simulink library "libbha_kinetic_cc"  (R2013b)
settings: Solver=FixedStepDiscrete  StartTime=0.0  StopTime=Inf  FixedStep=0.004  RelTol=1e-3
PostLoadFcn:
  | , if any(exist('dsrtsu_mdlpostloadfcn', 'file') == [2, 3, 6]), try dsrtsu_mdlpostloadfcn('Execute', bdroot); catch fprintf('Error in PostLoadFcn (dsrtsu_mdlpostloadfcn) for model "%s":\n %s\n', bdroot, lasterr); end, end,
libraries: libbha_parts_bellows x2
(part 3 of 4)

== matlab function libbha_kinetic_cc/lib_kinm_ext ==
  data: q input size=[9,1]; dq input size=[9,1]; H_1b_w input size=[4,4]; PAR_ell_ib input size=[3,1]; PAR_ell_ih input size=[3,1]; PAR_r_Bi input size=[3,1]; H_1h_w output size=[4,4]; H_2h_w output size=[4,4]; H_3h_w output size=[4,4]; dHdq_1h_w output size=[36,4]; dHdq_2h_w output size=[36,4]; dHdq_3h_w output size=[36,4]; dHPdq_1h_w output size=[36,4]; dHPdq_2h_w output size=[36,4]; dHPdq_3h_w output size=[36,4]; r_Bik_1h output size=[4,3]; r_Bik_2h output size=[4,3]; r_Bik_3h output size=[4,3]
% Kinetic Simulation
function [H_1h_w, H_2h_w, H_3h_w, dHdq_1h_w, dHdq_2h_w, dHdq_3h_w, dHPdq_1h_w, dHPdq_2h_w, dHPdq_3h_w, r_Bik_1h, r_Bik_2h, r_Bik_3h] =  ksim_ext(q,dq, H_1b_w, PAR_ell_ib, PAR_ell_ih, PAR_r_Bi)

  
    
    % Änderungen zut alten Version:
    % - Rückrechnung mit Offsets der 4. Dimension der Homogenen Transformation (HOxx)
    % - richtige Saturierung des Ausgangsdrucks (optional)
    % - Tensordarstellung vermieden (Vektoren oder Matrizen sofern möglich), daher auch mehr getrennte Variablen
    % - Zusammenfassung bei Berechnungen unter Ausnutzung von 0-Einträgen (schwerer lesbar und weniger allgemein, dafür schneller zu rechnen)


%% Zustands- und Ableitungsberechnung der Homogenen Transformationen
    
    k                 = [ calc_k_i(q(1), q(2), q(3), PAR_r_Bi(1));
                          calc_k_i(q(4), q(5), q(6), PAR_r_Bi(2));
                          calc_k_i(q(7), q(8), q(9), PAR_r_Bi(3)) ];
    
    dkdq_S1              = calc_dkdq_i(q(1), q(2), q(3), PAR_r_Bi(1));
    dkdq_S2              = calc_dkdq_i(q(4), q(5), q(6), PAR_r_Bi(2));
    dkdq_S3              = calc_dkdq_i(q(7), q(8), q(9), PAR_r_Bi(3));
	
	d2kdqdq_S1 	  = calc_d2kdqdq_i(q(1), q(2), q(3), PAR_r_Bi(1));
	d2kdqdq_S2 	  = calc_d2kdqdq_i(q(4), q(5), q(6), PAR_r_Bi(2));
	d2kdqdq_S3 	  = calc_d2kdqdq_i(q(7), q(8), q(9), PAR_r_Bi(3));
    
    % Relative Homogene Transformation und dessen Ableitung im lokalen Sektions-KoSy    
	[H_1h_1b, H_1b1, H_1h1] = calc_H_ih_ib(k(1), k(2), k(3), PAR_ell_ib(1), PAR_ell_ih(1));
    [H_2h_2b, H_2b2, H_2h2] = calc_H_ih_ib(k(4), k(5), k(6), PAR_ell_ib(2), PAR_ell_ih(2));
    [H_3h_3b, H_3b3, H_3h3] = calc_H_ih_ib(k(7), k(8), k(9), PAR_ell_ib(3), PAR_ell_ih(3));
    
    [dHdq_1h_1b, dHdk_1h_1b] = calc_dHdq_ih_ib(k(1), k(2), k(3), dkdq_S1, H_1b1, H_1h1);
    [dHdq_2h_2b, dHdk_2h_2b] = calc_dHdq_ih_ib(k(4), k(5), k(6), dkdq_S2, H_2b2, H_2h2);
    [dHdq_3h_3b, dHdk_3h_3b] = calc_dHdq_ih_ib(k(7), k(8), k(9), dkdq_S3, H_3b3, H_3h3);
	
   %[d2Hdqdq_1h_1b, d2Hdkdk_1h_1b] = calc_d2Hdqdq_ih_ib(k(1), k(2), k(3), dkdq_S1, d2kdqdq_S1, dHdk_1h_1b, H_1b1, H_1h1);
   %[d2Hdqdq_2h_2b, d2Hdkdk_2h_2b] = calc_d2Hdqdq_ih_ib(k(4), k(5), k(6), dkdq_S2, d2kdqdq_S2, dHdk_2h_2b, H_2b2, H_2h2);
   %[d2Hdqdq_3h_3b, d2Hdkdk_3h_3b] = calc_d2Hdqdq_ih_ib(k(7), k(8), k(9), dkdq_S3, d2kdqdq_S3, dHdk_3h_3b, H_3b3, H_3h3);
    [d2Hdqdq_1h_1b, ~            ] = calc_d2Hdqdq_ih_ib(k(1), k(2), k(3), dkdq_S1, d2kdqdq_S1, dHdk_1h_1b, H_1b1, H_1h1);
	[d2Hdqdq_2h_2b, ~            ] = calc_d2Hdqdq_ih_ib(k(4), k(5), k(6), dkdq_S2, d2kdqdq_S2, dHdk_2h_2b, H_2b2, H_2h2);
	[d2Hdqdq_3h_3b, ~            ] = calc_d2Hdqdq_ih_ib(k(7), k(8), k(9), dkdq_S3, d2kdqdq_S3, dHdk_3h_3b, H_3b3, H_3h3);
    
    % Absolute Homogene Transformation und dessen Ableitung im Welt-KoSy
    H_1h_w = H_1b_w * H_1h_1b;
    H_2h_w = H_1h_w * H_2h_2b;
    H_3h_w = H_2h_w * H_3h_3b; 
    
    dHdq_1h_w = zeros(4*9,4); % 4x4 Matrix abgeleitet nach 9 Zuständen q_i. H1 nach Zuständen 4..9 ist 0.
    dHdq_2h_w = zeros(4*9,4); % 4x4 Matrix abgeleitet nach 9 Zuständen q_i. H2 nach Zuständen 7..9 ist 0.
    dHdq_3h_w = zeros(4*9,4); % 4x4 Matrix abgeleitet nach 9 Zuständen q_i. 
    dHdq_1h_w((1:12)   ,:) = MM(H_1b_w,dHdq_1h_1b);
    dHdq_2h_w((1:12)   ,:) = MM(dHdq_1h_w(1:12,:),H_2h_2b);
    dHdq_2h_w((1:12)+12,:) = MM(H_1h_w,dHdq_2h_2b);
    dHdq_3h_w((1:24)   ,:) = MM(dHdq_2h_w(1:24,:),H_3h_3b);
    dHdq_3h_w((1:12)+24,:) = MM(H_2h_w,dHdq_3h_3b);
	
	d2Hdqdq_1h_w = zeros(4*9,4*9);
	d2Hdqdq_2h_w = zeros(4*9,4*9);
	d2Hdqdq_3h_w = zeros(4*9,4*9);
	d2Hdqdq_1h_w((1:12)   ,(1:12)   ) = MM(H_1b_w, d2Hdqdq_1h_1b);
	d2Hdqdq_2h_w((1:12)   ,(1:12)   ) = MM(d2Hdqdq_1h_w(1:12,1:12), H_2h_2b); % Quadrat innen
	d2Hdqdq_2h_w((1:12)   ,(1:4 )+12) = MM(dHdq_1h_w(1:12,:), dHdq_2h_2b(1:4 ,:)); % Blöcke Spalte rechts
	d2Hdqdq_2h_w((1:12)   ,(5:8 )+12) = MM(dHdq_1h_w(1:12,:), dHdq_2h_2b(5:8 ,:));
	d2Hdqdq_2h_w((1:12)   ,(9:12)+12) = MM(dHdq_1h_w(1:12,:), dHdq_2h_2b(9:12,:));
	d2Hdqdq_2h_w((1:12)+12,(1:12)+12) = MM(H_1h_w, d2Hdqdq_2h_2b); % Block Diagonal
	d2Hdqdq_2h_w((1:12)+12,(1:12)   ) = transpose4x4(d2Hdqdq_2h_w(1:12,(1:12)+12)); % Blöcke Zeile unten
	d2Hdqdq_3h_w((1:24)   ,(1:24)   ) = MM(d2Hdqdq_2h_w(1:24,1:24), H_3h_3b); % Quadrat innen
	d2Hdqdq_3h_w((1:24)   ,(1:4 )+24) = MM(dHdq_2h_w(1:24,:), dHdq_3h_3b(1:4 ,:)); % Blöcke Spalte rechts
	d2Hdqdq_3h_w((1:24)   ,(5:8 )+24) = MM(dHdq_2h_w(1:24,:), dHdq_3h_3b(5:8 ,:));
	d2Hdqdq_3h_w((1:24)   ,(9:12)+24) = MM(dHdq_2h_w(1:24,:), dHdq_3h_3b(9:12,:));
	d2Hdqdq_3h_w((1:12)+24,(1:12)+24) = MM(H_2h_w, d2Hdqdq_3h_3b); % Block Diagonal
	d2Hdqdq_3h_w((1:12)+24,(1:24)   ) = transpose4x4(d2Hdqdq_3h_w(1:24,(1:12)+24)); % Blöcke Zeile unten
	
	% Funktionen der Zeitableitung (HP)
	%HP_1h_w = calc_HP(dHdq_1h_w, dq); %zeros(4*9,4);
	%HP_2h_w = calc_HP(dHdq_2h_w, dq);
	%HP_3h_w = calc_HP(dHdq_3h_w, dq);
	
	dHPdq_1h_w = calc_dHPdq(d2Hdqdq_1h_w, dq); %zeros(4*9,4);
	dHPdq_2h_w = calc_dHPdq(d2Hdqdq_2h_w, dq);
	dHPdq_3h_w = calc_dHPdq(d2Hdqdq_3h_w, dq);
	
%% Kinetische Vorwärtsrechnung

    %r_S1_1h = [0;0;0;1];
    %r_S2_2h = [0;0;0;1];
    %r_S3_3h = [0;0;0;1];
    
    r_Bik_1h = [ PAR_r_Bi(1), -PAR_r_Bi(1)/2,         -PAR_r_Bi(1)/2;
				 0,            sqrt(3)/2*PAR_r_Bi(1),  -sqrt(3)/2*PAR_r_Bi(1)  
                 0, 0, 0; 1, 1, 1 ];
    r_Bik_2h = [ PAR_r_Bi(2), -PAR_r_Bi(2)/2,         -PAR_r_Bi(2)/2;
				 0,            sqrt(3)/2*PAR_r_Bi(2),  -sqrt(3)/2*PAR_r_Bi(2)  
                 0, 0, 0; 1, 1, 1 ];
    r_Bik_3h = [ PAR_r_Bi(3), -PAR_r_Bi(3)/2,         -PAR_r_Bi(3)/2;
				 0,            sqrt(3)/2*PAR_r_Bi(3),  -sqrt(3)/2*PAR_r_Bi(3)  
                 0, 0, 0; 1, 1, 1 ];

end

% ##################### Hilfsfunktionen #####################

%%  Konfigurationszustand k = [phi, kappa, ell]^T 

%  Konfigurationszustand einer Sektion 
function [k_i] = calc_k_i(q1,q2,q3, d)
    % Input:
    %   - qi = [ell_i1, ell_i2, ell_i3]^T       Aktorzustand
    %   - d                                     Radialer Abstand der Aktorsymmetrielinie  
    %
    % Output:
    %   - ki   [3 x 1]                          Konfigurationszustand 

    % Vermeidung Singularität
    qist_eps  = 1e-15;
    qist      = q1.^2 + q2.^2 + q3.^2 - q1.*q2 - q1.*q3 - q2.*q3;
    while (qist<qist_eps)
        q1      = q1 - 5e-8;
        qist  = q1.^2 + q2.^2 + q3.^2 - q1.*q2 - q1.*q3 - q2.*q3;
    end

    % Substitutionen
    q_sum   = q1 + q2 + q3;
    
    % Konfigurationszustand
    mphi    = atan2(sqrt(0.3e1) * (q3-q2) , (q2+q3 - 2*q1));
    mkappa  = 2.0 * sqrt(qist) / (d*q_sum);
    mell    = (q1 + q2 + q3)/3.0;
    
    k_i = [mphi;
           mkappa;
           mell];
end

% Partielle Ableitung 1. Ordnung nach q
function [dkdq_i] = calc_dkdq_i(q1,q2,q3, d)

    % Input:
	%   - qi = [ell_i1, ell_i2, ell_i3]^T       Aktorzustand
    %   - d                                     Radialer Abstand der Aktorsymmetrielinie
	%
	% Output:
	%   - dkdq_i   [3 x 3]                      Partielle Ableitung von Konfigurationszuständen ki nach Aktorzuständen qi 
 
    % Vermeidung Singularität
    qist_eps  = 1e-15;
    qist      = q1.^2 + q2.^2 + q3.^2 - q1.*q2 - q1.*q3 - q2.*q3;
    while (qist<qist_eps)
        q1      = q1-5e-8;
        qist  = q1.^2 + q2.^2 + q3.^2 - q1*q2 - q1*q3 - q2*q3;
    end

    % Substitutionen
    q_sum   = q1 + q2 + q3;

    % Ableitungen
    dkdq_i = zeros(3, 3);
    
    % dk1_dqb
    mdphi_dq1 =  sqrt(3.0) * ( q3 - q2) / qist / 2.0;
    mdphi_dq2 =  sqrt(3.0) * (-q3 + q1) / qist / 2.0;
    mdphi_dq3 = -sqrt(3.0) * (-q2 + q1) / qist / 2.0;
    
    dkdq_i(1, :) = [mdphi_dq1, mdphi_dq2, mdphi_dq3];
    
    % dk2_dqb
    mdkappa_dq1 =  3 * ( q2*q1 - q2^2  + q3*q1 - q3^2) / sqrt(qist) / d / q_sum^2;
    mdkappa_dq2 = -3 * (-q2*q1 - q2*q3 + q3^2  + q1^2) / sqrt(qist) / d / q_sum^2;
    mdkappa_dq3 = -3 * ( q2^2  - q2*q3 - q3*q1 + q1^2) / sqrt(qist) / d / q_sum^2;
    
    dkdq_i(2, :) = [mdkappa_dq1, mdkappa_dq2, mdkappa_dq3];
    
    % dk3_dqb
    mdell_dq1 = 1.0/3.0;
    mdell_dq2 = 1.0/3.0;
    mdell_dq3 = 1.0/3.0;
    
    dkdq_i(3, :) = [mdell_dq1, mdell_dq2, mdell_dq3];
end

function [d2kdqdq_i] = calc_d2kdqdq_i(q1,q2,q3, d)
% Input:
%   - qi = [ell_i1, ell_i2, ell_i3]^T       Aktorzustand
%
% Output:
%   - d2kdqdq_S1   [3*dim_qi x dim_qi]   Partielle Ableitung 2.Ord. von allen Konfigurationszuständen ki nach allen Aktorzuständen qi 
 
    % Vermeidung Singularität
    q_dist_eps  = 1e-15;
    q_dist      = q1 ^ 2 + q2 ^ 2 + q3 ^ 2 - q1 * q2 - q1 * q3 - q2 * q3;
    while (q_dist<q_dist_eps)
        q1      = q1-5e-8;
        q_dist  = q1 ^ 2 + q2 ^ 2 + q3 ^ 2 - q1 * q2 - q1 * q3 - q2 * q3;
    end

    % Substitutionen
    q_sum   = q1 + q2 + q3;

    % Ableitungen
    d2kdqdq_i = zeros(3*3, 3);
    
    % d2k1_dqbdqc
    mddphi_dq1dq1 = -sqrt(0.3e1) * (q3 - q2) / q_dist ^ 2 * (-q2 - q3 + 2 * q1) / 0.2e1;
    mddphi_dq1dq2 = -sqrt(0.3e1) * (-q2 ^ 2 + 2 * q2 * q3 - 2 * q3 * q1 + q1 ^ 2) / q_dist ^ 2 / 0.2e1;
    mddphi_dq1dq3 = sqrt(0.3e1) * (2 * q2 * q3 - 2 * q2 * q1 - q3 ^ 2 + q1 ^ 2) / q_dist ^ 2 / 0.2e1;
    
    mddphi_dq2dq1 = mddphi_dq1dq2;
    mddphi_dq2dq2 = sqrt(0.3e1) * (-q3 + q1) * (-2 * q2 + q3 + q1) / q_dist ^ 2 / 0.2e1;
    mddphi_dq2dq3 = -sqrt(0.3e1) * (q2 ^ 2 - 2 * q2 * q1 - q3 ^ 2 + 2 * q3 * q1) / q_dist ^ 2 / 0.2e1;
    
    mddphi_dq3dq1 = mddphi_dq1dq3;
    mddphi_dq3dq2 = mddphi_dq2dq3;
    mddphi_dq3dq3 = -sqrt(0.3e1) * (-q2 + q1) * (q2 - 2 * q3 + q1) / q_dist ^ 2 / 0.2e1;
    
    d2kdqdq_i([1, 4, 7], 1) = [mddphi_dq1dq1, mddphi_dq2dq1, mddphi_dq3dq1];
    d2kdqdq_i([1, 4, 7], 2) = [mddphi_dq1dq2, mddphi_dq2dq2, mddphi_dq3dq2];
    d2kdqdq_i([1, 4, 7], 3) = [mddphi_dq1dq3, mddphi_dq2dq3, mddphi_dq3dq3];
    
    % dk2_dqbdqc
    mddkappa_dq1dq1 = -0.3e1 / 0.2e1 * (-6 * q2 * q1 ^ 2 * q3 + 6 * q2 * q1 * q3 ^ 2 + 6 * q2 ^ 2 * q1 * q3 - 9 * q2 ^ 2 * q1 ^ 2 - 5 * q2 ^ 4 - 5 * q3 ^ 4 + 4 * q3 ^ 3 * q2 + 6 * q2 ^ 3 * q1 + 4 * q2 * q1 ^ 3 + 4 * q2 ^ 3 * q3 - 6 * q2 ^ 2 * q3 ^ 2 - 9 * q3 ^ 2 * q1 ^ 2 + 6 * q3 ^ 3 * q1 + 4 * q3 * q1 ^ 3) * (q_dist ^ (-0.3e1 / 0.2e1)) / d / (q_sum ^ 3);
    mddkappa_dq1dq2 = 0.3e1 / 0.2e1 * (2 * q2 ^ 4 + 3 * q3 ^ 4 + 3 * q2 * q1 ^ 2 * q3 + 3 * q2 ^ 2 * q1 * q3 - 3 * q2 * q1 * q3 ^ 2 + 6 * q2 ^ 2 * q1 ^ 2 - 7 * q2 ^ 3 * q1 - 7 * q2 * q1 ^ 3 - 3 * q2 ^ 3 * q3 + 9 * q2 ^ 2 * q3 ^ 2 - 3 * q3 * q1 ^ 3 + 9 * q3 ^ 2 * q1 ^ 2 - 7 * q3 ^ 3 * q2 - 7 * q3 ^ 3 * q1 + 2 * q1 ^ 4) * (q_dist ^ (-0.3e1 / 0.2e1)) / d / (q_sum ^ 3);
    mddkappa_dq1dq3 = 0.3e1 / 0.2e1 * (3 * q2 ^ 4 + 2 * q3 ^ 4 + 3 * q2 * q1 ^ 2 * q3 - 3 * q2 ^ 2 * q1 * q3 + 3 * q2 * q1 * q3 ^ 2 + 9 * q2 ^ 2 * q1 ^ 2 - 7 * q2 ^ 3 * q1 - 3 * q2 * q1 ^ 3 - 7 * q2 ^ 3 * q3 + 9 * q2 ^ 2 * q3 ^ 2 - 7 * q3 * q1 ^ 3 + 6 * q3 ^ 2 * q1 ^ 2 - 3 * q3 ^ 3 * q2 - 7 * q3 ^ 3 * q1 + 2 * q1 ^ 4) * (q_dist ^ (-0.3e1 / 0.2e1)) / d / (q_sum ^ 3);
    
    mddkappa_dq2dq1 = mddkappa_dq1dq2;
    mddkappa_dq2dq2 = 0.3e1 / 0.2e1 * (5 * q3 ^ 4 - 6 * q2 * q1 ^ 2 * q3 + 6 * q2 ^ 2 * q1 * q3 - 6 * q2 * q1 * q3 ^ 2 + 9 * q2 ^ 2 * q1 ^ 2 - 4 * q2 ^ 3 * q1 - 6 * q2 * q1 ^ 3 - 4 * q2 ^ 3 * q3 + 9 * q2 ^ 2 * q3 ^ 2 - 4 * q3 * q1 ^ 3 + 6 * q3 ^ 2 * q1 ^ 2 - 6 * q3 ^ 3 * q2 - 4 * q3 ^ 3 * q1 + 5 * q1 ^ 4) * (q_dist ^ (-0.3e1 / 0.2e1)) / d / (q_sum ^ 3);
    mddkappa_dq2dq3 = 0.3e1 / 0.2e1 * (2 * q2 ^ 4 + 2 * q3 ^ 4 - 3 * q2 * q1 ^ 2 * q3 + 3 * q2 ^ 2 * q1 * q3 + 3 * q2 * q1 * q3 ^ 2 + 9 * q2 ^ 2 * q1 ^ 2 - 3 * q2 ^ 3 * q1 - 7 * q2 ^ 3 * q3 + 6 * q2 ^ 2 * q3 ^ 2 - 7 * q2 * q3 ^ 3 - 3 * q3 ^ 3 * q1 + 9 * q3 ^ 2 * q1 ^ 2 - 7 * q1 ^ 3 * q3 - 7 * q1 ^ 3 * q2 + 3 * q1 ^ 4) * (q_dist ^ (-0.3e1 / 0.2e1)) / d / (q_sum ^ 3);

    mddkappa_dq3dq1 = mddkappa_dq1dq3;
    mddkappa_dq3dq2 = mddkappa_dq2dq3;
    mddkappa_dq3dq3 = 0.3e1 / 0.2e1 * (5 * q2 ^ 4 - 6 * q2 * q1 ^ 2 * q3 - 6 * q2 ^ 2 * q1 * q3 + 6 * q2 * q1 * q3 ^ 2 + 6 * q2 ^ 2 * q1 ^ 2 - 4 * q2 ^ 3 * q1 - 6 * q2 ^ 3 * q3 + 9 * q2 ^ 2 * q3 ^ 2 - 4 * q2 * q3 ^ 3 - 4 * q3 ^ 3 * q1 + 9 * q3 ^ 2 * q1 ^ 2 - 6 * q1 ^ 3 * q3 - 4 * q1 ^ 3 * q2 + 5 * q1 ^ 4) * (q_dist ^ (-0.3e1 / 0.2e1)) / d / (q_sum ^ 3);

    d2kdqdq_i([2, 5, 8], 1) = [mddkappa_dq1dq1, mddkappa_dq2dq1, mddkappa_dq3dq1];
    d2kdqdq_i([2, 5, 8], 2) = [mddkappa_dq1dq2, mddkappa_dq2dq2, mddkappa_dq3dq2];
    d2kdqdq_i([2, 5, 8], 3) = [mddkappa_dq1dq3, mddkappa_dq2dq3, mddkappa_dq3dq3];
    
    % dk3_dqbdqc
    % partielle Ableitungen 2. Ord von ell sind alle 0
end

%%  Homogene Transformationen 

%  Homogene Transformation 
%function [H_ih_ib] = calc_H_ih_ib(k1, k2, k3, PAR_ell_ib, PAR_ell_ih) 
function [H_ih_ib, H_im1_ib, H_ih_i] = calc_H_ih_ib(k1, k2, k3, PAR_ell_ib, PAR_ell_ih) 
    % Input:
    %   - ki = [phi, kappa, ell]^T              Konfigurationszustand
    %
    % Output:
    %   - H_i_im1   [4 x 4]                     Homogene Transformation
    
    % Vermeidung Singularität
    k2_eps = 1e-6;
    k2     = max([k2_eps, k2]);
    
    % Substitutionen
    sk1     = sin(k1);
    ck1     = cos(k1);
    sk2k3   = sin(k2 * k3);
    ck2k3   = cos(k2 * k3);
    
    % Trafo
    mHT_i_im1_11 = ck1 ^ 2 * (ck2k3 - 0.1e1) + 0.1e1;
    mHT_i_im1_12 = sk1 * ck1 * (ck2k3 - 0.1e1);
    mHT_i_im1_13 = ck1 * sk2k3;
    mHT_i_im1_14 = -ck1 * (ck2k3 - 0.1e1) / k2;
    
    mHT_i_im1_21 = sk1 * ck1 * (ck2k3 - 0.1e1);
    mHT_i_im1_22 = -ck1 ^ 2 * (ck2k3 - 0.1e1) + ck2k3;
    mHT_i_im1_23 = sk1 * sk2k3;
    mHT_i_im1_24 = -sk1 * (ck2k3 - 0.1e1) / k2;
    
    mHT_i_im1_31 = -ck1 * sk2k3;
    mHT_i_im1_32 = -sk1 * sk2k3;
    mHT_i_im1_33 = ck2k3;
    mHT_i_im1_34 = sk2k3 / k2;
    
    H_i_im1 = [mHT_i_im1_11, mHT_i_im1_12, mHT_i_im1_13, mHT_i_im1_14;
               mHT_i_im1_21, mHT_i_im1_22, mHT_i_im1_23, mHT_i_im1_24;
               mHT_i_im1_31, mHT_i_im1_32, mHT_i_im1_33, mHT_i_im1_34;
               0,            0,            0,            1            ];
           
    % Statische Begrenzungen
    H_im1_ib = eye(4);    
    H_ih_i   = eye(4);
    H_im1_ib(3,4) = PAR_ell_ib;
	H_ih_i(3,4)   = PAR_ell_ih;
    
    H_ih_ib = H_im1_ib * H_i_im1 * H_ih_i;
end

function [dHdk_i_i] = calc_dHdk_i_i(k1, k2, k3)
    % Input:
	%   - ki = [phi, kappa, ell]^T              Konfigurationszustand
	%
	% Output:
	%   - dH_i_in_im1_dka   [4*3x4]      Partielle Ableitung von H_i_in_im1 nach allen Konfigurationszuständen ki mit dim_ki=3
    
    % Vermeidung Singularität
    k2_eps = 1e-6;
    k2     = max([k2_eps, k2]);
    
    % Substitutionen
    sk1     = sin(k1);
    ck1     = cos(k1);
    sk2k3   = sin(k2 * k3);
    ck2k3   = cos(k2 * k3);
    
    dHdk_i_i = zeros(4*3, 4);
    
    % dHdk1_i_im1
    mdH_i_in_im1_dk1_11 = -2 * sk1 * ck1 * (ck2k3 - 1);
    mdH_i_in_im1_dk1_12 = 2 * ck2k3 * ck1 ^ 2 - ck2k3 - 2 * ck1 ^ 2 + 1;
    mdH_i_in_im1_dk1_13 = -sk1 * sk2k3;
    mdH_i_in_im1_dk1_14 = sk1 * (ck2k3 - 1) / k2;
    
    mdH_i_in_im1_dk1_21 = 2 * ck2k3 * ck1 ^ 2 - ck2k3 - 2 * ck1 ^ 2 + 1;
    mdH_i_in_im1_dk1_22 = 2 * sk1 * ck1 * (ck2k3 - 1);
    mdH_i_in_im1_dk1_23 = ck1 * sk2k3;
    mdH_i_in_im1_dk1_24 = -ck1 * (ck2k3 - 1) / k2;
    
    mdH_i_in_im1_dk1_31 = sk1 * sk2k3;
    mdH_i_in_im1_dk1_32 = -ck1 * sk2k3;
    mdH_i_in_im1_dk1_33 = 0;
    mdH_i_in_im1_dk1_34 = 0;
    
    dHdk_i_i(1:3,:) =         [mdH_i_in_im1_dk1_11, mdH_i_in_im1_dk1_12, mdH_i_in_im1_dk1_13, mdH_i_in_im1_dk1_14;
                               mdH_i_in_im1_dk1_21, mdH_i_in_im1_dk1_22, mdH_i_in_im1_dk1_23, mdH_i_in_im1_dk1_24;
                               mdH_i_in_im1_dk1_31, mdH_i_in_im1_dk1_32, mdH_i_in_im1_dk1_33, mdH_i_in_im1_dk1_34 ];
    
    % dHdk2_i_im1
    mdH_i_in_im1_dk2_11 = -ck1 ^ 2 * sk2k3 * k3;
    mdH_i_in_im1_dk2_12 = -sk1 * ck1 * sk2k3 * k3;
    mdH_i_in_im1_dk2_13 = ck1 * ck2k3 * k3;
    mdH_i_in_im1_dk2_14 = ck1 * (sk2k3 * k3 * k2 + ck2k3 - 1) / k2 ^ 2;
    
    mdH_i_in_im1_dk2_21 = -sk1 * ck1 * sk2k3 * k3;
    mdH_i_in_im1_dk2_22 = -sk2k3 * sk1 ^ 2 * k3;
    mdH_i_in_im1_dk2_23 = sk1 * ck2k3 * k3;
    mdH_i_in_im1_dk2_24 = sk1 * (sk2k3 * k3 * k2 + ck2k3 - 1) / k2 ^ 2;
    
    mdH_i_in_im1_dk2_31 = -ck1 * ck2k3 * k3;
    mdH_i_in_im1_dk2_32 = -sk1 * ck2k3 * k3;
    mdH_i_in_im1_dk2_33 = -sk2k3 * k3;
    mdH_i_in_im1_dk2_34 = (ck2k3 * k3 * k2 - sk2k3) / k2 ^ 2;
    
    dHdk_i_i(5:7,:) =         [mdH_i_in_im1_dk2_11, mdH_i_in_im1_dk2_12, mdH_i_in_im1_dk2_13, mdH_i_in_im1_dk2_14;
                               mdH_i_in_im1_dk2_21, mdH_i_in_im1_dk2_22, mdH_i_in_im1_dk2_23, mdH_i_in_im1_dk2_24;
                               mdH_i_in_im1_dk2_31, mdH_i_in_im1_dk2_32, mdH_i_in_im1_dk2_33, mdH_i_in_im1_dk2_34 ];
    
    % dHdk3_i_im1
    mdH_i_in_im1_dk3_11 = -ck1 ^ 2 * sk2k3 * k2;
    mdH_i_in_im1_dk3_12 = -sk1 * ck1 * sk2k3 * k2;
    mdH_i_in_im1_dk3_13 = ck1 * ck2k3 * k2;
    mdH_i_in_im1_dk3_14 = ck1 * sk2k3;
    
    mdH_i_in_im1_dk3_21 = -sk1 * ck1 * sk2k3 * k2;
    mdH_i_in_im1_dk3_22 = -sk2k3 * sk1 ^ 2 * k2;
    mdH_i_in_im1_dk3_23 = sk1 * ck2k3 * k2;
    mdH_i_in_im1_dk3_24 = sk1 * sk2k3;
    
    mdH_i_in_im1_dk3_31 = -ck1 * ck2k3 * k2;
    mdH_i_in_im1_dk3_32 = -sk1 * ck2k3 * k2;
    mdH_i_in_im1_dk3_33 = -sk2k3 * k2;
    mdH_i_in_im1_dk3_34 = ck2k3;
    
    dHdk_i_i(9:11,:) =        [mdH_i_in_im1_dk3_11, mdH_i_in_im1_dk3_12, mdH_i_in_im1_dk3_13, mdH_i_in_im1_dk3_14;
                               mdH_i_in_im1_dk3_21, mdH_i_in_im1_dk3_22, mdH_i_in_im1_dk3_23, mdH_i_in_im1_dk3_24;
                               mdH_i_in_im1_dk3_31, mdH_i_in_im1_dk3_32, mdH_i_in_im1_dk3_33, mdH_i_in_im1_dk3_34 ];
end

%function [dHdq_ih_ib, dHdk_ih_ib] = calc_dHdq_ih_ib(k1, k2, k3, dkdq_i, PAR_ell_ib, PAR_ell_ih)
function [dHdq_ih_ib, dHdk_ih_ib] = calc_dHdq_ih_ib(k1, k2, k3, dkdq_i, H_ibi, H_ihi)

    % Input:
	%   - ki = [phi, kappa, ell]^T              Konfigurationszustand
	%   - dkdq_i            [3=dim_kix3=dim_qi] Partielle Ableitung von allen Konfigurationszuständen ki nach allen Aktorzuständen qi 
	%
	% Output:
	%   - dH_i_in_im1_dqa   [4*3x4]      Partielle Ableitung von H_ih_ib nach allen Aktorzuständen qi mit dim_di = 3

    dHdq_ih_ib = zeros(4*3,4);

    % Statische Begrenzungen
    %H_im1_ib = eye(4);    
    %H_ih_i   = eye(4);
    %H_im1_ib(3,4) = PAR_ell_ib;
	%H_ih_i(3,4)   = PAR_ell_ih;
    
    % Kettenregel
    dHdk_ih_ib = calc_dHdk_i_i(k1, k2, k3);
    for j=1:3
		jm = j-1;
		%dHdq_ih_ib((1:4)+jm*4,:) = H_im1_ib * (dHdk_ih_ib(1:4,:).*dkdq_i(1,j) + dHdk_ih_ib(5:8,:).*dkdq_i(2,j) + dHdk_ih_ib(9:12,:).*dkdq_i(3,j)) * H_ih_i; % H_base * ( dHdq_i_i ) * H_head // mit dHdq_i_i = dH/dk1 * dk1/dqj + dH/dk2 * dk2/dqj + dH/dk3 * dk3/dqj
		dHdq_ih_ib((1:4)+jm*4,:) = H_ibi * (dHdk_ih_ib(1:4,:).*dkdq_i(1,j) + dHdk_ih_ib(5:8,:).*dkdq_i(2,j) + dHdk_ih_ib(9:12,:).*dkdq_i(3,j)) * H_ihi; % H_base * ( dHdq_i_i ) * H_head // mit dHdq_i_i = dH/dk1 * dk1/dqj + dH/dk2 * dk2/dqj + dH/dk3 * dk3/dqj
    end
end

function d2Hdkdk_ih_ib = calc_d2Hdkdk_ih_ib(k1, k2, k3)
% Input:
%   - ki = [phi, kappa, ell]^T              Konfigurationszustand
%
% Output
%   - d2Hdkdk_ih_ib   [4*dim_ki x 4*dim_ki]       Partielle Ableitung 2.Ord von H_i_in_im1 nach allen Konfigurationszuständen ki 
    
    % Vermeidung Singularität
    k2_eps = 1e-6;
    k2     = max([k2_eps, k2]);
    
    % Substitutionen
    sk1     = sin(k1);
    ck1     = cos(k1);
    sk2k3   = sin(k2 * k3);
    ck2k3   = cos(k2 * k3);
    
    dim_ki = 3;
    d2Hdkdk_ih_ib = zeros(4*dim_ki, 4*dim_ki);
    
% d2H_i_in_im1_dk1dk1
    mddH_i_in_im1_dk1dk1_11 = -0.4e1 * ck2k3 * ck1 ^ 2 + 0.2e1 * ck2k3 + 0.4e1 * ck1 ^ 2 - 0.2e1;
    mddH_i_in_im1_dk1dk1_12 = -0.4e1 * sk1 * ck1 * (ck2k3 - 0.1e1);
    mddH_i_in_im1_dk1dk1_13 = -ck1 * sk2k3;
    mddH_i_in_im1_dk1dk1_14 = ck1 * (ck2k3 - 0.1e1) / k2;
    
    mddH_i_in_im1_dk1dk1_21 = -0.4e1 * sk1 * ck1 * (ck2k3 - 0.1e1);
    mddH_i_in_im1_dk1dk1_22 = 0.4e1 * ck2k3 * ck1 ^ 2 - 0.2e1 * ck2k3 - 0.4e1 * ck1 ^ 2 + 0.2e1;
    mddH_i_in_im1_dk1dk1_23 = -sk1 * sk2k3;
    mddH_i_in_im1_dk1dk1_24 = sk1 * (ck2k3 - 0.1e1) / k2;
    
    mddH_i_in_im1_dk1dk1_31 = ck1 * sk2k3;
    mddH_i_in_im1_dk1dk1_32 = sk1 * sk2k3;
    mddH_i_in_im1_dk1dk1_33 = 0;
    mddH_i_in_im1_dk1dk1_34 = 0;
    
    d2Hdkdk_ih_ib(1:3, 1:4)       = [mddH_i_in_im1_dk1dk1_11, mddH_i_in_im1_dk1dk1_12, mddH_i_in_im1_dk1dk1_13, mddH_i_in_im1_dk1dk1_14;
                                           mddH_i_in_im1_dk1dk1_21, mddH_i_in_im1_dk1dk1_22, mddH_i_in_im1_dk1dk1_23, mddH_i_in_im1_dk1dk1_24;
                                           mddH_i_in_im1_dk1dk1_31, mddH_i_in_im1_dk1dk1_32, mddH_i_in_im1_dk1dk1_33, mddH_i_in_im1_dk1dk1_34 ]; 
    
    
    % d2H_i_in_im1_dk2dk2
    mddH_i_in_im1_dk2dk2_11 = -ck1 ^ 2 * ck2k3 * k3 ^ 2;
    mddH_i_in_im1_dk2dk2_12 = -sk1 * ck1 * ck2k3 * k3 ^ 2;
    mddH_i_in_im1_dk2dk2_13 = -ck1 * sk2k3 * k3 ^ 2;
    mddH_i_in_im1_dk2dk2_14 = -ck1 * (-ck2k3 * k3 ^ 2 * k2 ^ 2 + 0.2e1 * sk2k3 * k3 * k2 + 0.2e1 * ck2k3 - 0.2e1) / k2 ^ 3;
    
    mddH_i_in_im1_dk2dk2_21 = -sk1 * ck1 * ck2k3 * k3 ^ 2;
    mddH_i_in_im1_dk2dk2_22 = -ck2k3 * k3 ^ 2 * sk1 ^ 2;
    mddH_i_in_im1_dk2dk2_23 = -sk1 * sk2k3 * k3 ^ 2;
    mddH_i_in_im1_dk2dk2_24 = -sk1 * (-ck2k3 * k3 ^ 2 * k2 ^ 2 + 0.2e1 * sk2k3 * k3 * k2 + 0.2e1 * ck2k3 - 0.2e1) / k2 ^ 3;
    
    mddH_i_in_im1_dk2dk2_31 = ck1 * sk2k3 * k3 ^ 2;
    mddH_i_in_im1_dk2dk2_32 = sk1 * sk2k3 * k3 ^ 2;
    mddH_i_in_im1_dk2dk2_33 = -ck2k3 * k3 ^ 2;
    mddH_i_in_im1_dk2dk2_34 = -(sk2k3 * k3 ^ 2 * k2 ^ 2 + 0.2e1 * ck2k3 * k3 * k2 - 0.2e1 * sk2k3) / k2 ^ 3;
    
    d2Hdkdk_ih_ib(5:7, 5:8)       = [mddH_i_in_im1_dk2dk2_11, mddH_i_in_im1_dk2dk2_12, mddH_i_in_im1_dk2dk2_13, mddH_i_in_im1_dk2dk2_14;
                                           mddH_i_in_im1_dk2dk2_21, mddH_i_in_im1_dk2dk2_22, mddH_i_in_im1_dk2dk2_23, mddH_i_in_im1_dk2dk2_24;
                                           mddH_i_in_im1_dk2dk2_31, mddH_i_in_im1_dk2dk2_32, mddH_i_in_im1_dk2dk2_33, mddH_i_in_im1_dk2dk2_34 ]; 
                                       
    % d2H_i_in_im1_dk3dk3
    mddH_i_in_im1_dk3dk3_11 = -ck1 ^ 2 * ck2k3 * k2 ^ 2;
    mddH_i_in_im1_dk3dk3_12 = -sk1 * ck1 * ck2k3 * k2 ^ 2;
    mddH_i_in_im1_dk3dk3_13 = -ck1 * sk2k3 * k2 ^ 2;
    mddH_i_in_im1_dk3dk3_14 = ck1 * ck2k3 * k2;
    
    mddH_i_in_im1_dk3dk3_21 = -sk1 * ck1 * ck2k3 * k2 ^ 2;
    mddH_i_in_im1_dk3dk3_22 = -ck2k3 * k2 ^ 2 * sk1 ^ 2;
    mddH_i_in_im1_dk3dk3_23 = -sk1 * sk2k3 * k2 ^ 2;
    mddH_i_in_im1_dk3dk3_24 = sk1 * ck2k3 * k2;
    
    mddH_i_in_im1_dk3dk3_31 = ck1 * sk2k3 * k2 ^ 2;
    mddH_i_in_im1_dk3dk3_32 = sk1 * sk2k3 * k2 ^ 2;
    mddH_i_in_im1_dk3dk3_33 = -ck2k3 * k2 ^ 2;
    mddH_i_in_im1_dk3dk3_34 = -sk2k3 * k2;
    
    d2Hdkdk_ih_ib(9:11, 9:12)     = [mddH_i_in_im1_dk3dk3_11, mddH_i_in_im1_dk3dk3_12, mddH_i_in_im1_dk3dk3_13, mddH_i_in_im1_dk3dk3_14;
                                           mddH_i_in_im1_dk3dk3_21, mddH_i_in_im1_dk3dk3_22, mddH_i_in_im1_dk3dk3_23, mddH_i_in_im1_dk3dk3_24;
                                           mddH_i_in_im1_dk3dk3_31, mddH_i_in_im1_dk3dk3_32, mddH_i_in_im1_dk3dk3_33, mddH_i_in_im1_dk3dk3_34 ]; 
                                       
    % d2H_i_in_im1_dk1dk2 = d2H_i_in_im1_dk2dk1
    mddH_i_in_im1_dk1dk2_11 = 0.2e1 * sk1 * ck1 * sk2k3 * k3;
    mddH_i_in_im1_dk1dk2_12 = -sk2k3 * k3 * (0.2e1 * ck1 ^ 2 - 0.1e1);
    mddH_i_in_im1_dk1dk2_13 = -sk1 * ck2k3 * k3;
    mddH_i_in_im1_dk1dk2_14 = -sk1 * (sk2k3 * k3 * k2 + ck2k3 - 0.1e1) / k2 ^ 2;
    
    mddH_i_in_im1_dk1dk2_21 = -sk2k3 * k3 * (0.2e1 * ck1 ^ 2 - 0.1e1);
    mddH_i_in_im1_dk1dk2_22 = -0.2e1 * sk1 * ck1 * sk2k3 * k3;
    mddH_i_in_im1_dk1dk2_23 = ck1 * ck2k3 * k3;
    mddH_i_in_im1_dk1dk2_24 = ck1 * (sk2k3 * k3 * k2 + ck2k3 - 0.1e1) / k2 ^ 2;
    
    mddH_i_in_im1_dk1dk2_31 = sk1 * ck2k3 * k3;
    mddH_i_in_im1_dk1dk2_32 = -ck1 * ck2k3 * k3;
    mddH_i_in_im1_dk1dk2_33 = 0;
    mddH_i_in_im1_dk1dk2_34 = 0;
    
    d2Hdkdk_ih_ib(1:3, 5:8)       = [mddH_i_in_im1_dk1dk2_11, mddH_i_in_im1_dk1dk2_12, mddH_i_in_im1_dk1dk2_13, mddH_i_in_im1_dk1dk2_14;
                                           mddH_i_in_im1_dk1dk2_21, mddH_i_in_im1_dk1dk2_22, mddH_i_in_im1_dk1dk2_23, mddH_i_in_im1_dk1dk2_24;
                                           mddH_i_in_im1_dk1dk2_31, mddH_i_in_im1_dk1dk2_32, mddH_i_in_im1_dk1dk2_33, mddH_i_in_im1_dk1dk2_34 ]; 
    d2Hdkdk_ih_ib(5:7, 1:4) = d2Hdkdk_ih_ib(1:3, 5:8);
    
    % d2H_i_in_im1_dk1dk3 = d2H_i_in_im1_dk3dk1
    mddH_i_in_im1_dk1dk3_11 = 0.2e1 * sk1 * ck1 * sk2k3 * k2;
    mddH_i_in_im1_dk1dk3_12 = -sk2k3 * k2 * (0.2e1 * ck1 ^ 2 - 0.1e1);
    mddH_i_in_im1_dk1dk3_13 = -sk1 * ck2k3 * k2;
    mddH_i_in_im1_dk1dk3_14 = -sk1 * sk2k3;
    
    mddH_i_in_im1_dk1dk3_21 = -sk2k3 * k2 * (0.2e1 * ck1 ^ 2 - 0.1e1);
    mddH_i_in_im1_dk1dk3_22 = -0.2e1 * sk1 * ck1 * sk2k3 * k2;
    mddH_i_in_im1_dk1dk3_23 = ck1 * ck2k3 * k2;
    mddH_i_in_im1_dk1dk3_24 = ck1 * sk2k3;
    
    mddH_i_in_im1_dk1dk3_31 = sk1 * ck2k3 * k2;
    mddH_i_in_im1_dk1dk3_32 = -ck1 * ck2k3 * k2;
    mddH_i_in_im1_dk1dk3_33 = 0;
    mddH_i_in_im1_dk1dk3_34 = 0;
    
    d2Hdkdk_ih_ib(1:3, 9:12)      = [mddH_i_in_im1_dk1dk3_11, mddH_i_in_im1_dk1dk3_12, mddH_i_in_im1_dk1dk3_13, mddH_i_in_im1_dk1dk3_14;
                                           mddH_i_in_im1_dk1dk3_21, mddH_i_in_im1_dk1dk3_22, mddH_i_in_im1_dk1dk3_23, mddH_i_in_im1_dk1dk3_24;
                                           mddH_i_in_im1_dk1dk3_31, mddH_i_in_im1_dk1dk3_32, mddH_i_in_im1_dk1dk3_33, mddH_i_in_im1_dk1dk3_34 ]; 
    d2Hdkdk_ih_ib(9:11, 1:4) = d2Hdkdk_ih_ib(1:3, 9:12);
    
    % d2H_i_in_im1_dk2dk3 = d2H_i_in_im1_dk3dk2
    mddH_i_in_im1_dk2dk3_11 = -ck1 ^ 2 * (ck2k3 * k3 * k2 + sk2k3);
    mddH_i_in_im1_dk2dk3_12 = -sk1 * ck1 * (ck2k3 * k3 * k2 + sk2k3);
    mddH_i_in_im1_dk2dk3_13 = ck1 * (-sk2k3 * k3 * k2 + ck2k3);
    mddH_i_in_im1_dk2dk3_14 = ck1 * ck2k3 * k3;
    
    mddH_i_in_im1_dk2dk3_21 = -sk1 * ck1 * (ck2k3 * k3 * k2 + sk2k3);
    mddH_i_in_im1_dk2dk3_22 = -sk1 ^ 2 * (ck2k3 * k3 * k2 + sk2k3);
    mddH_i_in_im1_dk2dk3_23 = sk1 * (-sk2k3 * k3 * k2 + ck2k3);
    mddH_i_in_im1_dk2dk3_24 = sk1 * ck2k3 * k3;
    
    mddH_i_in_im1_dk2dk3_31 = -ck1 * (-sk2k3 * k3 * k2 + ck2k3);
    mddH_i_in_im1_dk2dk3_32 = -sk1 * (-sk2k3 * k3 * k2 + ck2k3);
    mddH_i_in_im1_dk2dk3_33 = -ck2k3 * k3 * k2 - sk2k3;
    mddH_i_in_im1_dk2dk3_34 = -sk2k3 * k3;
    
    d2Hdkdk_ih_ib(5:7, 9:12)      = [mddH_i_in_im1_dk2dk3_11, mddH_i_in_im1_dk2dk3_12, mddH_i_in_im1_dk2dk3_13, mddH_i_in_im1_dk2dk3_14;
                                           mddH_i_in_im1_dk2dk3_21, mddH_i_in_im1_dk2dk3_22, mddH_i_in_im1_dk2dk3_23, mddH_i_in_im1_dk2dk3_24;
                                           mddH_i_in_im1_dk2dk3_31, mddH_i_in_im1_dk2dk3_32, mddH_i_in_im1_dk2dk3_33, mddH_i_in_im1_dk2dk3_34 ]; 
    d2Hdkdk_ih_ib(9:11, 5:8) = d2Hdkdk_ih_ib(5:7, 9:12);
end

%function [d2Hdqdq_ih_ib, d2Hdkdk_ih_ib] = calc_d2Hdqdq_ih_ib(k1, k2, k3, dkdq_i, d2kdqdq_i, dHdk_ih_ib)
function [d2Hdqdq_ih_ib, d2Hdkdk_ih_ib] = calc_d2Hdqdq_ih_ib(k1, k2, k3, dkdq_i, d2kdqdq_i, dHdk_ih_ib, H_ibi, H_ihi)
	% Input:
%   - dkdqb_i               [3 x 3]           Partielle Ableitung von allen Konfigurationszuständen ki nach allen Aktorzuständen qi 
%   - d2kdqdq_i             [3*3 x 3]         Partielle Ableitung 2.Ord von allen Konfigurationszuständen ki nach allen Aktorzuständen qi 
%   - dHdk_ih_ib            [4*3 x 4]         Partielle Ableitung von H_ih_ib nach allen Konfigurationszuständen ki 
%
% Output:
%   - d2Hdqdq_ih_ib         [4*3 x 4*3]       Partielle Ableitung 2.Ord von H_ih_ib nach allen Aktorzuständen qi 
%   - d2Hdkdk_ih_ib		    [4*3 x 4*3]       Partielle Ableitung 2.Ord von H_ih_ib nach allen Konfigurationszuständen ki 
    
	d2Hdkdk_ih_ib = calc_d2Hdkdk_ih_ib(k1, k2, k3);
    
    d2Hdqdq_ih_ib = zeros(4*3, 4*3);
    for a = 1:3 % dim_qi
        for b = 1:3 % dim_qi
            for xi = 1:3 % dim_ki
                for chi = 1:3 % dim_ki
                    d2Hdqdq_ih_ib((1:4)+4*(a-1), (1:4)+4*(b-1)) = d2Hdqdq_ih_ib((1:4)+4*(a-1), (1:4)+4*(b-1)) + d2Hdkdk_ih_ib((1:4)+4*(xi-1), (1:4)+4*(chi-1)) * dkdq_i(chi, b) * dkdq_i(xi, a);					
                end
                d2Hdqdq_ih_ib((1:4)+4*(a-1), (1:4)+4*(b-1))     = d2Hdqdq_ih_ib((1:4)+4*(a-1), (1:4)+4*(b-1)) + dHdk_ih_ib((1:4)+4*(xi-1), :) * d2kdqdq_i(xi+3*(a-1), b);
            end
        end
    end
	d2Hdqdq_ih_ib = MM(MM(H_ibi,d2Hdqdq_ih_ib),H_ihi);
end

function [dHdt] = calc_HP(dHdq, dqdt)
% Input:
%   - dHdq    [4*dim_qi x 4]      Partielle Ableitung von H nach allen Aktorzuständen qi 
%   - dqdt    [dim_qi x 1]        Zeitableitung von allen Aktorzuständen qi 
%
% Output:
%   - dHdt    [4 x 4]             Zeitableitung von H 
    
   	dim_qi = size(dqdt, 1); %dim_qi = size(dHdq, 1)/4;
	
    dHdt = zeros(4, 4);
    for xi = 1:dim_qi
        dHdt =  dHdt + dHdq((1:4)+4*(xi-1),:)*dqdt(xi);        
    end
end

function [dHPdq] = calc_dHPdq(d2Hdqdq, dqdt) % Partielle Ableitung der Zeitableitung von H
% Input:
%   - d2Hdqdq    [4*dim_qi x 4*dim_qi]   Partielle Ableitung 2.Ord von H nach allen Aktorzuständen qi 
%   - dqdt       [dim_qi x 1]            Zeitableitung von allen Aktorzuständen qi 
%
% Output:
%   - dHPdq       [4*dim_qi x 4]          Partielle Ableitung nach allen Aktorzuständen qi der Zeitableitung von H 
    
    dim_qi = size(dqdt, 1);
    
    dHPdq = zeros(4*dim_qi, 4);
    for a = 1:dim_qi
        for xi = 1:dim_qi
            dHPdq((1:4)+4*(a-1),:) = dHPdq((1:4)+4*(a-1),:)...
                                      +d2Hdqdq((1:4)+4*(a-1),(1:4)+4*(xi-1))*dqdt(xi);
        end
    end
end


%% Matrix Helpers

function [H_2_0] = MMM(H_1_0, H_2_1) % Multiple Matrix Multiplication (Tensormultiplikation) für 4x4 * 4x4xn oder 4x4xn * 4x4

    H1_d3 = size(H_1_0,3);
    H2_d3 = size(H_2_1,3);
    H_2_0 = zeros(4,4,max(H1_d3,H2_d3));
    
    if H1_d3 == H2_d3
        for i=1:H2_d3
            H_2_0(:,:,i) = H_1_0(:,:,i) * H_2_1(:,:,i);
        end
    elseif H1_d3 == 1 && H2_d3 > 1
        for i=1:H2_d3
            H_2_0(:,:,i) = H_1_0 * H_2_1(:,:,i);
        end
    elseif H1_d3 > 1 && H2_d3 == 1
        for i=1:H1_d3
            H_2_0(:,:,i) = H_1_0(:,:,i) * H_2_1;
        end
    else
        error('case not handled here');
    end
end

function [H_2_0] = MM(H_1_0, H_2_1) % Matrix Multiplikation für 4x4 * 4nzx4ns
	% Input:
	%   - Eine Matrix [4x4]
	%   - Eine Matrix [4*nz x 4*ns]
	%
	% Output:
	%   - H_2_in_0 [4*n x 4*ns] = H_1_in_0*H_2_in_1

	[nz1, ns1] = size(H_1_0);
	[nz2, ns2] = size(H_2_1);

	nz_max = max(nz1./4, nz2./4);
	ns_max = max(ns1./4, ns2./4);

	H_2_0 = zeros(4*nz_max, 4*ns_max);

	if (nz1+ns1) < (nz2+ns2)
		for zz = 1:nz_max
			for ss = 1:ns_max
				H_2_0((1:4)+4*(zz-1), (1:4)+4*(ss-1)) = H_1_0 * H_2_1((1:4)+4*(zz-1), (1:4)+4*(ss-1));
			end
		end
	else
		for zz = 1:nz_max
			for ss = 1:ns_max
				H_2_0((1:4)+4*(zz-1), (1:4)+4*(ss-1)) = H_1_0((1:4)+4*(zz-1), (1:4)+4*(ss-1)) * H_2_1;
			end
		end
	end
end

function At = transpose4x4(A)
	% Input:
	%   - A     [4*z x 4*s]
	%
	% Output:
	%   - At    [4*s x 4*z]
	%
	% Bsp:
	% A = [a11, a12, a13, a14, b11, b12, b13, b14
	%      a21, a22, a23, a24, b21, b22, b23, b24
	%      a31, a32, a33, a34, b31, b32, b33, b34
	%      a41, a42, a43, a44, b41, b42, b43, b44];
	%
	% At =[a11, a12, a13, a14 
	%      a21, a22, a23, a24 
	%      a31, a32, a33, a34 
	%      a41, a42, a43, a44
	%      b11, b12, b13, b14
	%      b21, b22, b23, b24
	%      b31, b32, b33, b34
	%      b41, b42, b43, b44];

	At = zeros(size(A))';
	dim_z = size(A, 1)/4;
	dim_s = size(A, 2)/4;

	for iz = 1:dim_z
		for is = 1:dim_s
			At((1:4)+4*(is-1), (1:4)+4*(iz-1)) = A((1:4)+4*(iz-1), (1:4)+4*(is-1));
		end
	end
end

== matlab function libbha_kinetic_cc/lib_kin_hom_ext ==
  data: dHdq_1h_w input size=[36,4]; dHdq_2h_w input size=[36,4]; C output size=[9,9]; dHdq_3h_w input size=[36,4]; dHPdq_1h_w input size=[36,4]; dHPdq_2h_w input size=[36,4]; dHPdq_3h_w input size=[36,4]; PAR_M_i input size=[3,1]
function C  = ksim_kin_C(dHdq_1h_w, dHdq_2h_w, dHdq_3h_w, dHPdq_1h_w, dHPdq_2h_w, dHPdq_3h_w, PAR_M_i)


%% Kinetische Vorwärtsrechnung
    
	% SI = ceil(max(linspace(1,9,9)'*ones(1,9),ones(9,1)*linspace(1,9,9))/3);
    SI = [1 1 1 2 2 2 3 3 3;1 1 1 2 2 2 3 3 3;1 1 1 2 2 2 3 3 3;2 2 2 2 2 2 3 3 3;2 2 2 2 2 2 3 3 3;2 2 2 2 2 2 3 3 3;3 3 3 3 3 3 3 3 3;3 3 3 3 3 3 3 3 3;3 3 3 3 3 3 3 3 3];
	C1  = zeros(9,9); C2  = zeros(9,9); C3  = zeros(9,9);
    
    for row = 1:9
		rm = row - 1;
        for col = 1:9
			cm = col - 1;
			C3(row,col) = dHPdq_3h_w((1:4)+4*cm,4)'*dHdq_3h_w((1:4)+4*rm,4); % *PAR_M_i(3) am Ende
            if SI(row,col) <= 2
				C2(row,col) = dHPdq_2h_w((1:4)+4*cm,4)'*dHdq_2h_w((1:4)+4*rm,4); % *PAR_M_i(2) am Ende
                if SI(row,col) <= 1
                    C1(row,col) = dHPdq_1h_w((1:4)+4*cm,4)'*dHdq_1h_w((1:4)+4*rm,4); % *PAR_M_i(1) am Ende
                end
            end
        end
    end
	C = C1*PAR_M_i(1)  + C2*PAR_M_i(2)  + C3*PAR_M_i(3);


end

== matlab function libbha_kinetic_cc/lib_kinm ==
  data: q input size=[9,1]; H_1b_w input size=[4,4]; PAR_ell_ib input size=[3,1]; PAR_ell_ih input size=[3,1]; PAR_r_Bi input size=[3,1]; H_1h_w output size=[4,4]; H_2h_w output size=[4,4]; H_3h_w output size=[4,4]; dHdq_1h_w output size=[36,4]; dHdq_2h_w output size=[36,4]; dHdq_3h_w output size=[36,4]; r_Bik_1h output size=[4,3]; r_Bik_2h output size=[4,3]; r_Bik_3h output size=[4,3]
function [H_1h_w, H_2h_w, H_3h_w, dHdq_1h_w, dHdq_2h_w, dHdq_3h_w, r_Bik_1h, r_Bik_2h, r_Bik_3h] =  ksim_kinematic( q, H_1b_w,PAR_ell_ib,PAR_ell_ih, PAR_r_Bi)


%% Zustands- und Ableitungsberechnung der Homogenen Transformationen
    
    k                 = [ calc_k_i(q(1), q(2), q(3), PAR_r_Bi(1));
                          calc_k_i(q(4), q(5), q(6), PAR_r_Bi(2));
                          calc_k_i(q(7), q(8), q(9), PAR_r_Bi(3)) ];
    
    dkdq_S1              = calc_dkdq_i(q(1), q(2), q(3), PAR_r_Bi(1));
    dkdq_S2              = calc_dkdq_i(q(4), q(5), q(6), PAR_r_Bi(2));
    dkdq_S3              = calc_dkdq_i(q(7), q(8), q(9), PAR_r_Bi(3));
    
    % Relative Homogene Transformation und dessen Ableitung im lokalen Sektions-KoSy    
	[H_1h_1b, H_1b1, H_1h1] = calc_H_ih_ib(k(1), k(2), k(3), PAR_ell_ib(1), PAR_ell_ih(1));
    [H_2h_2b, H_2b2, H_2h2] = calc_H_ih_ib(k(4), k(5), k(6), PAR_ell_ib(2), PAR_ell_ih(2));
    [H_3h_3b, H_3b3, H_3h3] = calc_H_ih_ib(k(7), k(8), k(9), PAR_ell_ib(3), PAR_ell_ih(3));
    
    [dHdq_1h_1b, ~] = calc_dHdq_ih_ib(k(1), k(2), k(3), dkdq_S1, H_1b1, H_1h1);
    [dHdq_2h_2b, ~] = calc_dHdq_ih_ib(k(4), k(5), k(6), dkdq_S2, H_2b2, H_2h2);
    [dHdq_3h_3b, ~] = calc_dHdq_ih_ib(k(7), k(8), k(9), dkdq_S3, H_3b3, H_3h3);
    
    % Absolute Homogene Transformation und dessen Ableitung im Welt-KoSy
    H_1h_w = H_1b_w * H_1h_1b;
    H_2h_w = H_1h_w * H_2h_2b;
    H_3h_w = H_2h_w * H_3h_3b; 
    
    dHdq_1h_w = zeros(4*9,4); % 4x4 Matrix abgeleitet nach 9 Zuständen q_i. H1 nach Zuständen 4..9 ist 0.
    dHdq_2h_w = zeros(4*9,4); % 4x4 Matrix abgeleitet nach 9 Zuständen q_i. H2 nach Zuständen 7..9 ist 0.
    dHdq_3h_w = zeros(4*9,4); % 4x4 Matrix abgeleitet nach 9 Zuständen q_i. 
    dHdq_1h_w((1:12)   ,:) = MM(H_1b_w,dHdq_1h_1b);
    dHdq_2h_w((1:12)   ,:) = MM(dHdq_1h_w(1:12,:),H_2h_2b);
    dHdq_2h_w((1:12)+12,:) = MM(H_1h_w,dHdq_2h_2b);
    dHdq_3h_w((1:24)   ,:) = MM(dHdq_2h_w(1:24,:),H_3h_3b);
    dHdq_3h_w((1:12)+24,:) = MM(H_2h_w,dHdq_3h_3b);
	
%% Kinetische Vorwärtsrechnung

    %r_S1_1h = [0;0;0;1];
    %r_S2_2h = [0;0;0;1];
    %r_S3_3h = [0;0;0;1];
    
    r_Bik_1h = [ PAR_r_Bi(1), -PAR_r_Bi(1)/2,         -PAR_r_Bi(1)/2;
				 0,            sqrt(3)/2*PAR_r_Bi(1),  -sqrt(3)/2*PAR_r_Bi(1)  
                 0, 0, 0; 1, 1, 1 ];
    r_Bik_2h = [ PAR_r_Bi(2), -PAR_r_Bi(2)/2,         -PAR_r_Bi(2)/2;
				 0,            sqrt(3)/2*PAR_r_Bi(2),  -sqrt(3)/2*PAR_r_Bi(2)  
                 0, 0, 0; 1, 1, 1 ];
    r_Bik_3h = [ PAR_r_Bi(3), -PAR_r_Bi(3)/2,         -PAR_r_Bi(3)/2;
				 0,            sqrt(3)/2*PAR_r_Bi(3),  -sqrt(3)/2*PAR_r_Bi(3)  
                 0, 0, 0; 1, 1, 1 ];

end

% ##################### Hilfsfunktionen #####################

%%  Konfigurationszustand k = [phi, kappa, ell]^T 

%  Konfigurationszustand einer Sektion 
function [k_i] = calc_k_i(q1,q2,q3, d)
    % Input:
    %   - qi = [ell_i1, ell_i2, ell_i3]^T       Aktorzustand
    %   - d                                     Radialer Abstand der Aktorsymmetrielinie  
    %
    % Output:
    %   - ki   [3 x 1]                          Konfigurationszustand 

    % Vermeidung Singularität
    qist_eps  = 1e-15;
    qist      = q1.^2 + q2.^2 + q3.^2 - q1.*q2 - q1.*q3 - q2.*q3;
    while (qist<qist_eps)
        q1      = q1 - 5e-8;
        qist  = q1.^2 + q2.^2 + q3.^2 - q1.*q2 - q1.*q3 - q2.*q3;
    end

    % Substitutionen
    q_sum   = q1 + q2 + q3;
    
    % Konfigurationszustand
    mphi    = atan2(sqrt(0.3e1) * (q3-q2) , (q2+q3 - 2*q1));
    mkappa  = 2.0 * sqrt(qist) / (d*q_sum);
    mell    = (q1 + q2 + q3)/3.0;
    
    k_i = [mphi;
           mkappa;
           mell];
end

% Partielle Ableitung 1. Ordnung nach q
function [dkdq_i] = calc_dkdq_i(q1,q2,q3, d)

    % Input:
	%   - qi = [ell_i1, ell_i2, ell_i3]^T       Aktorzustand
    %   - d                                     Radialer Abstand der Aktorsymmetrielinie
	%
	% Output:
	%   - dkdq_i   [3 x 3]                      Partielle Ableitung von Konfigurationszuständen ki nach Aktorzuständen qi 
 
    % Vermeidung Singularität
    qist_eps  = 1e-15;
    qist      = q1.^2 + q2.^2 + q3.^2 - q1.*q2 - q1.*q3 - q2.*q3;
    while (qist<qist_eps)
        q1      = q1-5e-8;
        qist  = q1.^2 + q2.^2 + q3.^2 - q1*q2 - q1*q3 - q2*q3;
    end

    % Substitutionen
    q_sum   = q1 + q2 + q3;

    % Ableitungen
    dkdq_i = zeros(3, 3);
    
    % dk1_dqb
    mdphi_dq1 =  sqrt(3.0) * ( q3 - q2) / qist / 2.0;
    mdphi_dq2 =  sqrt(3.0) * (-q3 + q1) / qist / 2.0;
    mdphi_dq3 = -sqrt(3.0) * (-q2 + q1) / qist / 2.0;
    
    dkdq_i(1, :) = [mdphi_dq1, mdphi_dq2, mdphi_dq3];
    
    % dk2_dqb
    mdkappa_dq1 =  3 * ( q2*q1 - q2^2  + q3*q1 - q3^2) / sqrt(qist) / d / q_sum^2;
    mdkappa_dq2 = -3 * (-q2*q1 - q2*q3 + q3^2  + q1^2) / sqrt(qist) / d / q_sum^2;
    mdkappa_dq3 = -3 * ( q2^2  - q2*q3 - q3*q1 + q1^2) / sqrt(qist) / d / q_sum^2;
    
    dkdq_i(2, :) = [mdkappa_dq1, mdkappa_dq2, mdkappa_dq3];
    
    % dk3_dqb
    mdell_dq1 = 1.0/3.0;
    mdell_dq2 = 1.0/3.0;
    mdell_dq3 = 1.0/3.0;
    
    dkdq_i(3, :) = [mdell_dq1, mdell_dq2, mdell_dq3];
end

%%  Homogene Transformationen 

%  Homogene Transformation 
%function [H_ih_ib] = calc_H_ih_ib(k1, k2, k3, PAR_ell_ib, PAR_ell_ih) 
function [H_ih_ib, H_im1_ib, H_ih_i] = calc_H_ih_ib(k1, k2, k3, PAR_ell_ib, PAR_ell_ih) 
    % Input:
    %   - ki = [phi, kappa, ell]^T              Konfigurationszustand
    %
    % Output:
    %   - H_i_im1   [4 x 4]                     Homogene Transformation
    
    % Vermeidung Singularität
    k2_eps = 1e-6;
    k2     = max([k2_eps, k2]);
    
    % Substitutionen
    sk1     = sin(k1);
    ck1     = cos(k1);
    sk2k3   = sin(k2 * k3);
    ck2k3   = cos(k2 * k3);
    
    % Trafo
    mHT_i_im1_11 = ck1 ^ 2 * (ck2k3 - 0.1e1) + 0.1e1;
    mHT_i_im1_12 = sk1 * ck1 * (ck2k3 - 0.1e1);
    mHT_i_im1_13 = ck1 * sk2k3;
    mHT_i_im1_14 = -ck1 * (ck2k3 - 0.1e1) / k2;
    
    mHT_i_im1_21 = sk1 * ck1 * (ck2k3 - 0.1e1);
    mHT_i_im1_22 = -ck1 ^ 2 * (ck2k3 - 0.1e1) + ck2k3;
    mHT_i_im1_23 = sk1 * sk2k3;
    mHT_i_im1_24 = -sk1 * (ck2k3 - 0.1e1) / k2;
    
    mHT_i_im1_31 = -ck1 * sk2k3;
    mHT_i_im1_32 = -sk1 * sk2k3;
    mHT_i_im1_33 = ck2k3;
    mHT_i_im1_34 = sk2k3 / k2;
    
    H_i_im1 = [mHT_i_im1_11, mHT_i_im1_12, mHT_i_im1_13, mHT_i_im1_14;
               mHT_i_im1_21, mHT_i_im1_22, mHT_i_im1_23, mHT_i_im1_24;
               mHT_i_im1_31, mHT_i_im1_32, mHT_i_im1_33, mHT_i_im1_34;
               0,            0,            0,            1            ];
           
    % Statische Begrenzungen
    H_im1_ib = eye(4);    
    H_ih_i   = eye(4);
    H_im1_ib(3,4) = PAR_ell_ib;
	H_ih_i(3,4)   = PAR_ell_ih;
    
    H_ih_ib = H_im1_ib * H_i_im1 * H_ih_i;
end

function [dHdk_i_i] = calc_dHdk_i_i(k1, k2, k3)
    % Input:
	%   - ki = [phi, kappa, ell]^T              Konfigurationszustand
	%
	% Output:
	%   - dH_i_in_im1_dka   [4*3x4]      Partielle Ableitung von H_i_in_im1 nach allen Konfigurationszuständen ki mit dim_ki=3
    
    % Vermeidung Singularität
    k2_eps = 1e-6;
    k2     = max([k2_eps, k2]);
    
    % Substitutionen
    sk1     = sin(k1);
    ck1     = cos(k1);
    sk2k3   = sin(k2 * k3);
    ck2k3   = cos(k2 * k3);
    
    dHdk_i_i = zeros(4*3, 4);
    
    % dHdk1_i_im1
    mdH_i_in_im1_dk1_11 = -2 * sk1 * ck1 * (ck2k3 - 1);
    mdH_i_in_im1_dk1_12 = 2 * ck2k3 * ck1 ^ 2 - ck2k3 - 2 * ck1 ^ 2 + 1;
    mdH_i_in_im1_dk1_13 = -sk1 * sk2k3;
    mdH_i_in_im1_dk1_14 = sk1 * (ck2k3 - 1) / k2;
    
    mdH_i_in_im1_dk1_21 = 2 * ck2k3 * ck1 ^ 2 - ck2k3 - 2 * ck1 ^ 2 + 1;
    mdH_i_in_im1_dk1_22 = 2 * sk1 * ck1 * (ck2k3 - 1);
    mdH_i_in_im1_dk1_23 = ck1 * sk2k3;
    mdH_i_in_im1_dk1_24 = -ck1 * (ck2k3 - 1) / k2;
    
    mdH_i_in_im1_dk1_31 = sk1 * sk2k3;
    mdH_i_in_im1_dk1_32 = -ck1 * sk2k3;
    mdH_i_in_im1_dk1_33 = 0;
    mdH_i_in_im1_dk1_34 = 0;
    
    dHdk_i_i(1:3,:) =         [mdH_i_in_im1_dk1_11, mdH_i_in_im1_dk1_12, mdH_i_in_im1_dk1_13, mdH_i_in_im1_dk1_14;
                               mdH_i_in_im1_dk1_21, mdH_i_in_im1_dk1_22, mdH_i_in_im1_dk1_23, mdH_i_in_im1_dk1_24;
                               mdH_i_in_im1_dk1_31, mdH_i_in_im1_dk1_32, mdH_i_in_im1_dk1_33, mdH_i_in_im1_dk1_34 ];
    
    % dHdk2_i_im1
    mdH_i_in_im1_dk2_11 = -ck1 ^ 2 * sk2k3 * k3;
    mdH_i_in_im1_dk2_12 = -sk1 * ck1 * sk2k3 * k3;
    mdH_i_in_im1_dk2_13 = ck1 * ck2k3 * k3;
    mdH_i_in_im1_dk2_14 = ck1 * (sk2k3 * k3 * k2 + ck2k3 - 1) / k2 ^ 2;
    
    mdH_i_in_im1_dk2_21 = -sk1 * ck1 * sk2k3 * k3;
    mdH_i_in_im1_dk2_22 = -sk2k3 * sk1 ^ 2 * k3;
    mdH_i_in_im1_dk2_23 = sk1 * ck2k3 * k3;
    mdH_i_in_im1_dk2_24 = sk1 * (sk2k3 * k3 * k2 + ck2k3 - 1) / k2 ^ 2;
    
    mdH_i_in_im1_dk2_31 = -ck1 * ck2k3 * k3;
    mdH_i_in_im1_dk2_32 = -sk1 * ck2k3 * k3;
    mdH_i_in_im1_dk2_33 = -sk2k3 * k3;
    mdH_i_in_im1_dk2_34 = (ck2k3 * k3 * k2 - sk2k3) / k2 ^ 2;
    
    dHdk_i_i(5:7,:) =         [mdH_i_in_im1_dk2_11, mdH_i_in_im1_dk2_12, mdH_i_in_im1_dk2_13, mdH_i_in_im1_dk2_14;
                               mdH_i_in_im1_dk2_21, mdH_i_in_im1_dk2_22, mdH_i_in_im1_dk2_23, mdH_i_in_im1_dk2_24;
                               mdH_i_in_im1_dk2_31, mdH_i_in_im1_dk2_32, mdH_i_in_im1_dk2_33, mdH_i_in_im1_dk2_34 ];
    
    % dHdk3_i_im1
    mdH_i_in_im1_dk3_11 = -ck1 ^ 2 * sk2k3 * k2;
    mdH_i_in_im1_dk3_12 = -sk1 * ck1 * sk2k3 * k2;
    mdH_i_in_im1_dk3_13 = ck1 * ck2k3 * k2;
    mdH_i_in_im1_dk3_14 = ck1 * sk2k3;
    
    mdH_i_in_im1_dk3_21 = -sk1 * ck1 * sk2k3 * k2;
    mdH_i_in_im1_dk3_22 = -sk2k3 * sk1 ^ 2 * k2;
    mdH_i_in_im1_dk3_23 = sk1 * ck2k3 * k2;
    mdH_i_in_im1_dk3_24 = sk1 * sk2k3;
    
    mdH_i_in_im1_dk3_31 = -ck1 * ck2k3 * k2;
    mdH_i_in_im1_dk3_32 = -sk1 * ck2k3 * k2;
    mdH_i_in_im1_dk3_33 = -sk2k3 * k2;
    mdH_i_in_im1_dk3_34 = ck2k3;
    
    dHdk_i_i(9:11,:) =        [mdH_i_in_im1_dk3_11, mdH_i_in_im1_dk3_12, mdH_i_in_im1_dk3_13, mdH_i_in_im1_dk3_14;
                               mdH_i_in_im1_dk3_21, mdH_i_in_im1_dk3_22, mdH_i_in_im1_dk3_23, mdH_i_in_im1_dk3_24;
                               mdH_i_in_im1_dk3_31, mdH_i_in_im1_dk3_32, mdH_i_in_im1_dk3_33, mdH_i_in_im1_dk3_34 ];
end

%function [dHdq_ih_ib, dHdk_ih_ib] = calc_dHdq_ih_ib(k1, k2, k3, dkdq_i, PAR_ell_ib, PAR_ell_ih)
function [dHdq_ih_ib, dHdk_ih_ib] = calc_dHdq_ih_ib(k1, k2, k3, dkdq_i, H_ibi, H_ihi)

    % Input:
	%   - ki = [phi, kappa, ell]^T              Konfigurationszustand
	%   - dkdq_i            [3=dim_kix3=dim_qi] Partielle Ableitung von allen Konfigurationszuständen ki nach allen Aktorzuständen qi 
	%
	% Output:
	%   - dH_i_in_im1_dqa   [4*3x4]      Partielle Ableitung von H_ih_ib nach allen Aktorzuständen qi mit dim_di = 3

    dHdq_ih_ib = zeros(4*3,4);

    % Statische Begrenzungen
    %H_im1_ib = eye(4);    
    %H_ih_i   = eye(4);
    %H_im1_ib(3,4) = PAR_ell_ib;
	%H_ih_i(3,4)   = PAR_ell_ih;
    
    % Kettenregel
    dHdk_ih_ib = calc_dHdk_i_i(k1, k2, k3);
    for j=1:3
		jm = j-1;
		%dHdq_ih_ib((1:4)+jm*4,:) = H_im1_ib * (dHdk_ih_ib(1:4,:).*dkdq_i(1,j) + dHdk_ih_ib(5:8,:).*dkdq_i(2,j) + dHdk_ih_ib(9:12,:).*dkdq_i(3,j)) * H_ih_i; % H_base * ( dHdq_i_i ) * H_head // mit dHdq_i_i = dH/dk1 * dk1/dqj + dH/dk2 * dk2/dqj + dH/dk3 * dk3/dqj
		dHdq_ih_ib((1:4)+jm*4,:) = H_ibi * (dHdk_ih_ib(1:4,:).*dkdq_i(1,j) + dHdk_ih_ib(5:8,:).*dkdq_i(2,j) + dHdk_ih_ib(9:12,:).*dkdq_i(3,j)) * H_ihi; % H_base * ( dHdq_i_i ) * H_head // mit dHdq_i_i = dH/dk1 * dk1/dqj + dH/dk2 * dk2/dqj + dH/dk3 * dk3/dqj
    end
end

%% Matrix Helpers

function [H_2_0] = MM(H_1_0, H_2_1) % Matrix Multiplikation für 4x4 * 4nzx4ns
	% Input:
	%   - Eine Matrix [4x4]
	%   - Eine Matrix [4*nz x 4*ns]
	%
	% Output:
	%   - H_2_in_0 [4*n x 4*ns] = H_1_in_0*H_2_in_1

	[nz1, ns1] = size(H_1_0);
	[nz2, ns2] = size(H_2_1);

	nz_max = max(nz1./4, nz2./4);
	ns_max = max(ns1./4, ns2./4);

	H_2_0 = zeros(4*nz_max, 4*ns_max);

	if (nz1+ns1) < (nz2+ns2)
		for zz = 1:nz_max
			for ss = 1:ns_max
				H_2_0((1:4)+4*(zz-1), (1:4)+4*(ss-1)) = H_1_0 * H_2_1((1:4)+4*(zz-1), (1:4)+4*(ss-1));
			end
		end
	else
		for zz = 1:nz_max
			for ss = 1:ns_max
				H_2_0((1:4)+4*(zz-1), (1:4)+4*(ss-1)) = H_1_0((1:4)+4*(zz-1), (1:4)+4*(ss-1)) * H_2_1;
			end
		end
	end
end

== matlab function libbha_kinetic_cc/lib_revkin_inhom_S1 ==
  data: H_1h_w input size=[4,4]; dHdq_1h_w input size=[12,4]; r_Bik_1h input size=[4,3]; rHinv output size=[3,3]; rH output size=[3,3]
function [rHinv, rH]   = ksim_rev_tinv(H_1h_w, dHdq_1h_w, r_Bik_1h)
% kinvsim_fav_4c

    % Herleitung: Review 2014
    % pd = 1/AP * Hinv * tau_d + pAmb
    % tau_d: Anteile der Mechanik-DGL (anteilig)
    

    %% Htilde
    
    HF11 = [H_1h_w(:,3)'*dHdq_1h_w( 1: 4,:)*r_Bik_1h(:,1), H_1h_w(:,3)'*dHdq_1h_w( 1: 4,:)*r_Bik_1h(:,2), H_1h_w(:,3)'*dHdq_1h_w( 1: 4,:)*r_Bik_1h(:,3) ;
            H_1h_w(:,3)'*dHdq_1h_w( 5: 8,:)*r_Bik_1h(:,1), H_1h_w(:,3)'*dHdq_1h_w( 5: 8,:)*r_Bik_1h(:,2), H_1h_w(:,3)'*dHdq_1h_w( 5: 8,:)*r_Bik_1h(:,3) ;
            H_1h_w(:,3)'*dHdq_1h_w( 9:12,:)*r_Bik_1h(:,1), H_1h_w(:,3)'*dHdq_1h_w( 9:12,:)*r_Bik_1h(:,2), H_1h_w(:,3)'*dHdq_1h_w( 9:12,:)*r_Bik_1h(:,3)   ];
        
    rHtilde = HF11;
    
    %% Hhat
    
    rHhat = eye(3);
    rHhatinv = eye(3);

    %% Zusammenführung
    rHinv = rHhat/rHtilde;
    rH = rHtilde*rHhatinv;

end

== matlab function libbha_kinetic_cc/lib_kin_hom_S1 ==
  data: H_1h_w input size=[4,4]; dHdq_1h_w input size=[12,4]; r_Bik_1h input size=[4,3]; g_w input size=[3,1]; delta_F_ik_Spring input size=[3,1]; delta_F_ik_Damper input size=[3,1]; delta_F_ik_Bending input size=[3,1]; PAR_M_i input size=1; B output size=[3,3]; Ns output size=[3,1]; Ng output size=[3,1]; Nb output size=[3,1]; Nd output size=[3,1]
function [B, Ns, Ng, Nb, Nd]  = ksim_kin_BN(H_1h_w, dHdq_1h_w, r_Bik_1h, g_w, delta_F_ik_Spring, delta_F_ik_Damper, delta_F_ik_Bending, PAR_M_i)
% kinvsim_fav_4b2
    
    % Änderungen zut alten Version:
    % - Rückrechnung mit Offsets der 4. Dimension der Homogenen Transformation (HOxx)
    % - richtige Saturierung des Ausgangsdrucks (optional)
    % - Tensordarstellung vermieden (Vektoren oder Matrizen sofern möglich), daher auch mehr getrennte Variablen
    % - Zusammenfassung bei Berechnungen unter Ausnutzung von 0-Einträgen (schwerer lesbar und weniger allgemein, dafür schneller zu rechnen)

    g_w4 = [g_w; 0];

%% Kraftdifferenz (passiv)

    F_Spring_d  = delta_F_ik_Spring;
    F_Damper_d  = delta_F_ik_Damper;
    F_Bending_d = delta_F_ik_Bending;
    
%% Kinetische Vorwärtsrechnung

	B1  = zeros(3,3); 
    N1g = zeros(3,1); 
    N1s = zeros(3,1); 
    N1d = zeros(3,1); 
    N1b = zeros(3,1); 
    
    for row = 1:3
		rm = row - 1;
        for col = 1:3
			cm = col - 1;
            B1(row,col) = dHdq_1h_w((1:4)+4*cm,4)'*dHdq_1h_w((1:4)+4*rm,4); % *PAR_M_i(1) am Ende
        end
        N1g(row) = - g_w4'*dHdq_1h_w((1:4)+4*rm,4); % *PAR_M_i(1) am Ende
        
        for bi=1:3  
            N1s(row) = N1s(row) + (H_1h_w(:,3)*F_Spring_d(bi))'  * dHdq_1h_w((1:4)+4*rm,:)*r_Bik_1h(:,bi);
            N1d(row) = N1d(row) + (H_1h_w(:,3)*F_Damper_d(bi))'  * dHdq_1h_w((1:4)+4*rm,:)*r_Bik_1h(:,bi);
            N1b(row) = N1b(row) + (H_1h_w(:,3)*F_Bending_d(bi))' * dHdq_1h_w((1:4)+4*rm,:)*r_Bik_1h(:,bi);
        end
    end
    
    B    = B1*PAR_M_i(1);
    Ng   = N1g*PAR_M_i(1);
    Ns   = N1s;
    Nd   = N1d;
    Nb   = N1b;

end

== matlab function libbha_kinetic_cc/lib_kin_hom_ext_S1 ==
  data: dHdq_1h_w input size=[12,4]; C output size=[3,3]; dHPdq_1h_w input size=[12,4]; PAR_M_i input size=1
function C  = ksim_kin_C(dHdq_1h_w, dHPdq_1h_w, PAR_M_i)


%% Kinetische Vorwärtsrechnung
    
	C1  = zeros(3,3); 
    
    for row = 1:3
		rm = row - 1;
        for col = 1:3
            cm = col - 1;
			C1(row,col) = dHPdq_1h_w((1:4)+4*cm,4)'*dHdq_1h_w((1:4)+4*rm,4); % *PAR_M_i(1) am Ende
        end
    end
	C = C1*PAR_M_i(1);


end
